simulink library "Valeo_Simulink_Library_EC"  (R2020b)
settings: Solver=ode45  StartTime=0.0  StopTime=10.0  RelTol=1e-3  EnableMultiTasking=on
undefined symbols (not defined in the file): A, B, C, Count_Max, D, InitValue, j, ke, kf, kt, L, Length, MaxIniVal, MaxVal, MinVal, NumBits1, NumBits2, P, p0, Q, R, Simulink_Library, Ts, x0
libraries: $bdroot x9, simulink x4, fixpt_dtprop x4
(part 3 of 4)

== system Valeo_Simulink_Library_EC/Signal_Operations/PosHys ==
  High : Inport
  In : Inport  Port=2
  Low : Inport  Port=3
  DataTypeDuplicate : DataTypeDuplicate  NumInputPorts=3
  Hysteresis : Subsystem  Description=Hysteresis  RTWFileName=sal_math
      settings: RTWSystemCode=Inline  RTWFcnNameOpts=Use subsystem name  RTWFileNameOpts=User specified
  UnitDelay : UnitDelay  SampleTime=-1  HasFrameUpgradeWarning=on
  Out : Outport  VectorParamsAs1DForOutWhenUnconnected=off
  wires:
  Hysteresis/1(Out) -> Out/1, UnitDelay/1
  UnitDelay/1 -> Hysteresis/4(RemainderIN)
  Low/1 -> DataTypeDuplicate/3, Hysteresis/1(Low)
  In/1 -> DataTypeDuplicate/2, Hysteresis/2(In)
  High/1 -> DataTypeDuplicate/1, Hysteresis/3(High)

== system Valeo_Simulink_Library_EC/Signal_Operations/RisingEdge ==
  In : Inport
  LogicalOperator : Logic  Tag=struct('inputs','2','comment',struct('text','','placement',1),'logdata',struct('maxnumvals',inf,'plotchannels',[],'loggingmode',3,'channels',1),'operator','AND','output',struct('variable','','description','','name','$S_$B','address','','class','default','type','Bool','unit',''),'scalingvalid',0,'date',733067.68458487268)  RequirementInfo={} %GIDa_46b4697c_c428_4231_8e35_ed6f95728904  OutDataTypeStr=boolean
  LogicalOperator1 : Logic  Tag=struct('inputs','1','comment',struct('text','','placement',1),'logdata',struct('maxnumvals',inf,'plotchannels',[],'loggingmode',3,'channels',1),'operator','NOT','output',struct('variable','','description','','name','$S_$B','address','','class','default','type','Bool','unit',''),'scalingvalid',0,'date',733067.68458533566)  Operator=NOT  Inputs=1  OutDataTypeStr=boolean
  UnitDelay : UnitDelay  RequirementInfo={} %GIDa_e97586d9_635f_41d8_ab1f_7563d0e0a8e3  InitialCondition=Init  SampleTime=-1  HasFrameUpgradeWarning=on
  Out : Outport  OutDataTypeStr=boolean  VectorParamsAs1DForOutWhenUnconnected=off
  wires:
  UnitDelay/1 -> LogicalOperator/2
  LogicalOperator1/1 -> UnitDelay/1
  LogicalOperator/1 -> Out/1
  In/1 -> LogicalOperator/1, LogicalOperator1/1

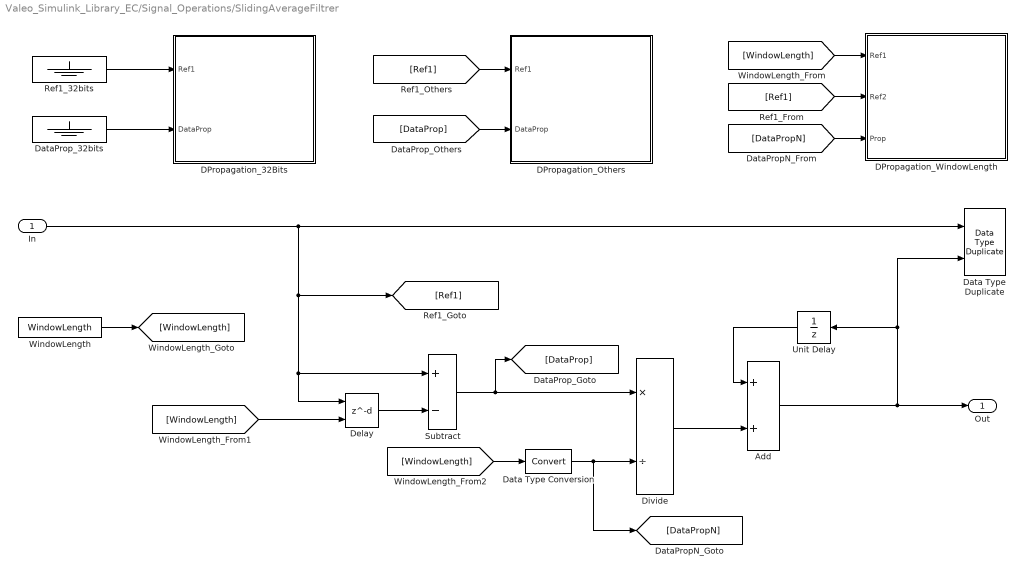
== system Valeo_Simulink_Library_EC/Signal_Operations/SlidingAverageFiltrer ==
  In : Inport
  Add : Sum  OutDataTypeStr=Inherit: Inherit via back propagation  RndMeth=Nearest  SaturateOnIntegerOverflow=on
  DPropagation_32Bits : Subsystem
  DPropagation_Others : Subsystem
  DPropagation_WindowLength : Subsystem
  Data Type Duplicate : DataTypeDuplicate
  Data Type Conversion : DataTypeConversion
  DataProp_32bits : Ground
  Delay : Delay  DelayLengthSource=Input port  DelayLength=Length  DelayLengthUpperLimit=WindowLength  InitialCondition=0
      settings: InputPortMap=u0,p1
  Divide : Product  Inputs=*/  RndMeth=Nearest  OutDataTypeStr=Inherit: Same as first input
  Ref1_32bits : Ground
  Subtract : Sum  Inputs=+-  OutDataTypeStr=Inherit: Inherit via back propagation  RndMeth=Nearest  SaturateOnIntegerOverflow=on
  Unit Delay : UnitDelay  SampleTime=-1  HasFrameUpgradeWarning=on
  WindowLength : Constant  Value=WindowLength  OutDataTypeStr=Inherit: Inherit via back propagation  SampleTime=-1
  Out : Outport  VectorParamsAs1DForOutWhenUnconnected=off
  wires:
  Add/1 -> Out/1, Unit Delay/1, Data Type Duplicate/2
  Delay/1 -> Subtract/2
  Divide/1 -> Add/2
  Unit Delay/1 -> Add/1
  In/1 -> [Ref1], Subtract/1, Delay/1, Data Type Duplicate/1
  Subtract/1 -> [DataProp], Divide/1
  [Ref1] -> DPropagation_Others/1(Ref1)
  [DataProp] -> DPropagation_Others/2(DataProp)
  Ref1_32bits/1 -> DPropagation_32Bits/1(Ref1)
  DataProp_32bits/1 -> DPropagation_32Bits/2(DataProp)
  WindowLength/1 -> [WindowLength]
  [WindowLength] -> Delay/2
  [WindowLength] -> Data Type Conversion/1
  [WindowLength] -> DPropagation_WindowLength/1(Ref1)
  [Ref1] -> DPropagation_WindowLength/2(Ref2)
  Data Type Conversion/1 -> [DataPropN], Divide/2
  [DataPropN] -> DPropagation_WindowLength/3(Prop)

== system Valeo_Simulink_Library_EC/Signal_Operations/TurnOffDelay ==
  In : Inport
  Tdly : Inport  Port=2
  Te : Inport  Port=3
  CheckDly : RelationalOperator  Operator=<  OutDataTypeStr=boolean  RndMeth=Nearest  InputSameDT=on
  Check_Tdly_unsigned : fixpt_dtprop/Data Type Police Unsigned Only
      settings: SourceProductBaseCode=SL
  Check_Te_unsigned : fixpt_dtprop/Data Type Police Unsigned Only
      settings: SourceProductBaseCode=SL
  Divide : Product  Inputs=*/  OutDataTypeStr=uint32  RndMeth=Nearest  SaturateOnIntegerOverflow=on
  Inc : Constant  OutDataTypeStr=Inherit: Inherit via back propagation
  Increment : Sum  InputSameDT=on  OutDataTypeStr=Inherit: Inherit via back propagation  SaturateOnIntegerOverflow=on
  InitialCondition : Subsystem  Description=InitialCondition
  LogicalOperator : Logic  Operator=OR  AllPortsSameDT=off  OutDataTypeStr=boolean
  NewVal : UnitDelay  SampleTime=-1  HasFrameUpgradeWarning=on
  Reset : Constant  Value=0  OutDataTypeStr=Inherit: Inherit via back propagation
  ResetSwitch : Switch  Criteria=u2 ~= 0  InputSameDT=on
  StartDelay : UnitDelay  SampleTime=-1  HasFrameUpgradeWarning=on
  Out : Outport  VectorParamsAs1DForOutWhenUnconnected=off
  wires:
  LogicalOperator/1 -> Out/1
  Reset/1 -> ResetSwitch/1
  ResetSwitch/1 -> Increment/1, CheckDly/1
  Increment/1 -> NewVal/1
  CheckDly/1 -> LogicalOperator/1
  In/1 -> LogicalOperator/2, InitialCondition/1(CheckDir), StartDelay/1
  NewVal/1 -> InitialCondition/3(NewVal)
  InitialCondition/1(CalcVal) -> ResetSwitch/3
  StartDelay/1 -> ResetSwitch/2
  Divide/1 -> CheckDly/2, InitialCondition/2(Tdly)
  Te/1 -> Check_Te_unsigned/1, Divide/2
  Tdly/1 -> Check_Tdly_unsigned/1, Divide/1
  Inc/1 -> Increment/2

== system Valeo_Simulink_Library_EC/Signal_Operations/TurnOnDelay ==
  In : Inport
  Tdly : Inport  Port=2
  Te : Inport  Port=3
  CheckDly : RelationalOperator  OutDataTypeStr=boolean  RndMeth=Nearest  InputSameDT=on
  Check_Tdly_unsigned : fixpt_dtprop/Data Type Police Unsigned Only
      settings: SourceProductBaseCode=SL
  Check_Te_unsigned : fixpt_dtprop/Data Type Police Unsigned Only
      settings: SourceProductBaseCode=SL
  Divide : Product  Inputs=*/  OutDataTypeStr=uint32  SaturateOnIntegerOverflow=on
  Inc : Constant  OutDataTypeStr=Inherit: Inherit via back propagation
  Increment : Sum  InputSameDT=on  OutDataTypeStr=Inherit: Inherit via back propagation  RndMeth=Simplest  SaturateOnIntegerOverflow=on
  InitialCondition : Subsystem  Description=InitialCondition
  InitialDelayl : UnitDelay  InitialCondition=1  SampleTime=-1  HasFrameUpgradeWarning=on
  LogicalOperator : Logic  AllPortsSameDT=off  OutDataTypeStr=boolean
  NewVal : UnitDelay  SampleTime=-1  HasFrameUpgradeWarning=on
  Reset : Constant  Value=0  OutDataTypeStr=Inherit: Inherit via back propagation
  ResetSwitch : Switch  Criteria=u2 ~= 0  InputSameDT=on
  Out : Outport  VectorParamsAs1DForOutWhenUnconnected=off
  wires:
  InitialDelayl/1 -> ResetSwitch/2
  LogicalOperator/1 -> Out/1
  ResetSwitch/1 -> Increment/1, CheckDly/1
  Increment/1 -> NewVal/1
  CheckDly/1 -> LogicalOperator/1
  NewVal/1 -> InitialCondition/1(NewVal)
  In/1 -> LogicalOperator/2, InitialCondition/3(CheckDir), InitialDelayl/1
  InitialCondition/1(CalcVal) -> ResetSwitch/1
  Reset/1 -> ResetSwitch/3
  Tdly/1 -> Divide/1, Check_Tdly_unsigned/1
  Te/1 -> Divide/2, Check_Te_unsigned/1
  Divide/1 -> InitialCondition/2(Tdly), CheckDly/2
  Inc/1 -> Increment/2

== system Valeo_Simulink_Library_EC/Signal_Operations/VSL_ClarkTransformation_EC_Blk ==
  A : Inport  PortDimensions=1
  B : Inport  Port=2  PortDimensions=1
  C : Inport  Port=3  PortDimensions=1
  Calculation : Subsystem  Description=Calculations for clarke transfromation  RequirementInfo={} %GIDa_91c9902b_4297_47d8_bcc7_839692c95106
  datatype_protection : Subsystem  Description=forcing input and output to have the same data type  RequirementInfo={} %GIDa_ba0677aa_132e_4dc0_8af7_6cee4e109de7
  Alpha : Outport  RequirementInfo={} %GIDa_2f11082c_73d3_4ed4_8929_d03a8ab0ed51  PortDimensions=1  VectorParamsAs1DForOutWhenUnconnected=off
  Beta : Outport  RequirementInfo={} %GIDa_b2cc2919_a1d0_479c_944a_1162b348937b  Port=2  PortDimensions=1  VectorParamsAs1DForOutWhenUnconnected=off
  wires:
  B/1 -> [B]  "B"
  A/1 -> [A]  "A"
  C/1 -> [C]  "C"
  [A] -> Calculation/1(A)
  [B] -> Calculation/2(B)
  [C] -> Calculation/3(C)
  datatype_protection/1(Alpha) -> Alpha/1
  datatype_protection/2(Beta) -> Beta/1
  Calculation/1(Alpha) -> datatype_protection/1(Alpha_temp)
  Calculation/2(Beta) -> datatype_protection/2(Beta_temp)
  [A] -> datatype_protection/3(A)
  [B] -> datatype_protection/4(B)
  [C] -> datatype_protection/5(C)

== system Valeo_Simulink_Library_EC/Signal_Operations/VSL_InverseClarkTransformation_EC_Blk ==
  Alpha : Inport
  Beta : Inport  Port=2
  Calculations : Subsystem  Description=claclulations of Inverse clarke transform
  "DataTypeProtection " : Subsystem  Description=make sure all inputs and outputs have the same datatype
  A : Outport  VectorParamsAs1DForOutWhenUnconnected=off
  B : Outport  Port=2  VectorParamsAs1DForOutWhenUnconnected=off
  C : Outport  Port=3  VectorParamsAs1DForOutWhenUnconnected=off
  wires:
  Calculations/1(A) -> "DataTypeProtection "/1(A_t)
  Calculations/2(B) -> "DataTypeProtection "/2(B_t)
  Calculations/3(C) -> "DataTypeProtection "/3(C_t)
  "DataTypeProtection "/1(A) -> A/1
  "DataTypeProtection "/2(B) -> B/1
  "DataTypeProtection "/3(C) -> C/1
  [Alpha] -> Calculations/1(Alpha)
  [Beta] -> Calculations/2(Beta)
  [Alpha] -> "DataTypeProtection "/4(Alpha)
  [Beta] -> "DataTypeProtection "/5(Beta)
  Alpha/1 -> [Alpha]
  Beta/1 -> [Beta]

== system Valeo_Simulink_Library_EC/Signal_Operations/VSL_InverseParkTransformation_EC_Blk ==
  D : Inport
  Q : Inport  Port=2
  Sin : Inport  Port=3
  Cos : Inport  Port=4
  Calculation : Subsystem  Description=This Block is transforming dq axies with d axis aligned with Phase A into alpha-beta axises
      settings: RTWFcnNameOpts=Use subsystem name
  dataTypeProtection : Subsystem  Description=make sure inputs and outputs have the same data type
  Alpha : Outport  VectorParamsAs1DForOutWhenUnconnected=off
  Beta : Outport  Port=2  VectorParamsAs1DForOutWhenUnconnected=off
  wires:
  [Cos] -> dataTypeProtection/6(Cos)
  [Sin] -> dataTypeProtection/5(Sin)
  [Q] -> dataTypeProtection/4(Q)
  [D] -> dataTypeProtection/3(D)
  dataTypeProtection/1(Alpha) -> Alpha/1  "Alpha"
  dataTypeProtection/2(Beta) -> Beta/1  "Beta"
  [Cos] -> Calculation/3(cos)
  [Sin] -> Calculation/2(sin)
  Cos/1 -> [Cos]
  Sin/1 -> [Sin]
  [Q] -> Calculation/4(Q)
  [D] -> Calculation/1(D)
  D/1 -> [D]
  Q/1 -> [Q]
  Calculation/2(Beta) -> dataTypeProtection/2(beta_t)
  Calculation/1(Alpha) -> dataTypeProtection/1(alpha_t)

== system Valeo_Simulink_Library_EC/Signal_Operations/VSL_ParkTransformation_Blk ==
  Alpha : Inport
  Beta : Inport  Port=2
  Sin : Inport  Port=3
  Cos : Inport  Port=4
  Calculation : Subsystem  Description=This Block is transforming alpha-beta axises into dq axies with d axie aligned with Phase A
      settings: RTWSystemCode=Nonreusable function  RTWFcnNameOpts=Use subsystem name
  DataTypeProtection : Subsystem  Description=make sure all inputs and outputs have the sane data type
  D : Outport  VectorParamsAs1DForOutWhenUnconnected=off
  Q : Outport  Port=2  VectorParamsAs1DForOutWhenUnconnected=off
  wires:
  Beta/1 -> [beta]
  Alpha/1 -> [alpha]
  [alpha] -> Calculation/1(alpha)
  [beta] -> Calculation/4(beta)
  Calculation/1(d) -> DataTypeProtection/1(d_t)  "D"
  Calculation/2(q) -> DataTypeProtection/2(q_t)  "Q"
  Sin/1 -> [sin]
  Cos/1 -> [cos]
  [sin] -> Calculation/2(sin)
  [cos] -> Calculation/3(cos)
  DataTypeProtection/1(D) -> D/1
  DataTypeProtection/2(Q) -> Q/1
  [alpha] -> DataTypeProtection/3(Alpha)
  [beta] -> DataTypeProtection/4(Beta)
  [sin] -> DataTypeProtection/5(Sin)
  [cos] -> DataTypeProtection/6(Cos)

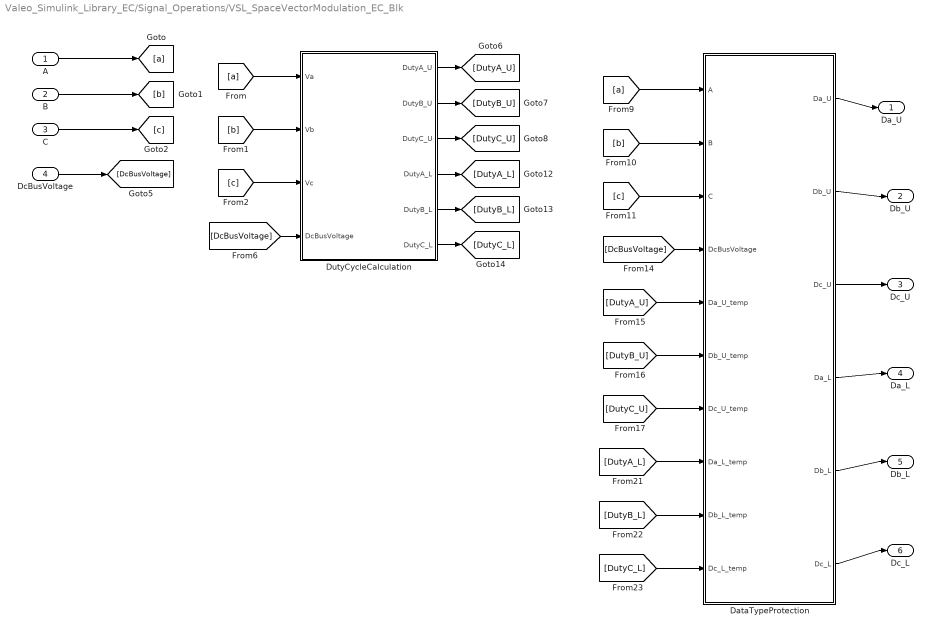
== system Valeo_Simulink_Library_EC/Signal_Operations/VSL_SpaceVectorModulation_EC_Blk ==
  A : Inport
  B : Inport  Port=2
  C : Inport  Port=3
  DcBusVoltage : Inport  Port=4
  DataTypeProtection : Subsystem  Description=applying the data type protection
  DutyCycleCalculation : Subsystem  Description=Calculate the duty cycle for every phase
  Da_U : Outport  VectorParamsAs1DForOutWhenUnconnected=off
  Db_U : Outport  Port=2  VectorParamsAs1DForOutWhenUnconnected=off
  Dc_U : Outport  Port=3  VectorParamsAs1DForOutWhenUnconnected=off
  Da_L : Outport  Port=4  VectorParamsAs1DForOutWhenUnconnected=off
  Db_L : Outport  Port=5  VectorParamsAs1DForOutWhenUnconnected=off
  Dc_L : Outport  Port=6  VectorParamsAs1DForOutWhenUnconnected=off
  wires:
  DataTypeProtection/6(Dc_L) -> Dc_L/1
  DataTypeProtection/5(Db_L) -> Db_L/1
  DataTypeProtection/4(Da_L) -> Da_L/1
  DataTypeProtection/3(Dc_U) -> Dc_U/1
  DataTypeProtection/2(Db_U) -> Db_U/1
  DataTypeProtection/1(Da_U) -> Da_U/1
  [DutyC_L] -> DataTypeProtection/10(Dc_L_temp)
  [DutyA_L] -> DataTypeProtection/8(Da_L_temp)
  [DutyB_L] -> DataTypeProtection/9(Db_L_temp)
  [DutyC_U] -> DataTypeProtection/7(Dc_U_temp)
  [DutyB_U] -> DataTypeProtection/6(Db_U_temp)
  DutyCycleCalculation/4(DutyA_L) -> [DutyA_L]
  DutyCycleCalculation/5(DutyB_L) -> [DutyB_L]
  DutyCycleCalculation/6(DutyC_L) -> [DutyC_L]
  [c] -> DutyCycleCalculation/3(Vc)
  [b] -> DutyCycleCalculation/2(Vb)
  [a] -> DutyCycleCalculation/1(Va)
  B/1 -> [b]
  C/1 -> [c]
  A/1 -> [a]
  DcBusVoltage/1 -> [DcBusVoltage]
  [DcBusVoltage] -> DutyCycleCalculation/4(DcBusVoltage)
  [a] -> DataTypeProtection/1(A)
  [b] -> DataTypeProtection/2(B)
  [c] -> DataTypeProtection/3(C)
  [DcBusVoltage] -> DataTypeProtection/4(DcBusVoltage)
  DutyCycleCalculation/1(DutyA_U) -> [DutyA_U]
  DutyCycleCalculation/2(DutyB_U) -> [DutyB_U]
  DutyCycleCalculation/3(DutyC_U) -> [DutyC_U]
  [DutyA_U] -> DataTypeProtection/5(Da_U_temp)

== system Valeo_Simulink_Library_EC/Utilities/EventToVar ==
  Evt : Inport
  Constant1 : Constant  Value=0  OutDataTypeStr=boolean  SampleTime=-1
  Constant2 : Constant  OutDataTypeStr=boolean  SampleTime=-1
  Function-Call Subsystem : Subsystem  Description=|  TreatAsAtomicUnit=on
      | Function-Call
      | Subsystem
  Logical Operator1 : Logic  Tag=AM,Std,Inputs,1;CMP,Operator,Inputs;  Operator=NOT  Inputs=1  AllPortsSameDT=off  OutDataTypeStr=boolean
  Relational Operator : RelationalOperator  Operator=~=  OutDataTypeStr=boolean  RndMeth=Nearest
  Switch : Switch  Criteria=u2 ~= 0
  Unit Delay1 : UnitDelay  SampleTime=-1  HasFrameUpgradeWarning=on
  Unit Delay2 : UnitDelay  SampleTime=-1  HasFrameUpgradeWarning=on
  Var : Outport  VectorParamsAs1DForOutWhenUnconnected=off
  wires:
  Logical Operator1/1 -> Relational Operator/1, Unit Delay1/1
  Switch/1 -> Var/1
  Relational Operator/1 -> Switch/2
  Constant1/1 -> Switch/3
  Constant2/1 -> Switch/1
  Unit Delay1/1 -> Relational Operator/2
  Function-Call Subsystem/1(out) -> Logical Operator1/1, Unit Delay2/1
  Unit Delay2/1 -> Function-Call Subsystem/1(in)
  Evt/1 -> Function-Call Subsystem/Trigger

== system Valeo_Simulink_Library_EC/Utilities/ScribeInfo ==

== system Valeo_Simulink_Library_EC/Math_Operations/VSL_DynamicSecureDivision_EC_Blk/Calculation ==
  Num : Inport  PortDimensions=1
  Den : Inport  Port=2  PortDimensions=1
  Positive_Inf : Inport  Port=3  PortDimensions=1
  Negative_Inf : Inport  Port=4  PortDimensions=1
  Nan : Inport  Port=5  PortDimensions=1
  ZeroBand_Den : Inport  Port=6  PortDimensions=1
  ZeroBand_Num : Inport  Port=7  PortDimensions=1
  DecisionLogic : Subsystem  Description=Decision logic for dynamic secure division. this block is performing secure division with Positive_inf, Negative_inf, Nan is dynamic in run time
  Divide : Subsystem  TreatAsAtomicUnit=on
  Merge : Merge  InitialOutput=0
  Output : Outport  VectorParamsAs1DForOutWhenUnconnected=off
  wires:
  ZeroBand_Num/1 -> DecisionLogic/7(ZeroBand_Num)
  ZeroBand_Den/1 -> DecisionLogic/6(ZeroBand_Den)
  Positive_Inf/1 -> DecisionLogic/3(Positive_Inf)
  Negative_Inf/1 -> DecisionLogic/4(Negative_Inf)
  Nan/1 -> DecisionLogic/5(Nan)
  DecisionLogic/1(Out) -> Merge/1
  DecisionLogic/2(Divide) -> Divide/Trigger
  Merge/1 -> Output/1
  Divide/1(output) -> Merge/2
  Den/1 -> DecisionLogic/2(Den), Divide/2(Den)
  Num/1 -> DecisionLogic/1(Num), Divide/1(Num)

== system Valeo_Simulink_Library_EC/Math_Operations/VSL_DynamicSecureDivision_EC_Blk/datatype_protection ==
  Output_Temp : Inport  PortDimensions=1
  P_inf : Inport  Port=2  PortDimensions=1
  N_inf : Inport  Port=3  PortDimensions=1
  Nan : Inport  Port=4  PortDimensions=1
  Den : Inport  Port=5  PortDimensions=1
  ZeroBand_Den : Inport  Port=6  PortDimensions=1
  Num : Inport  Port=7  PortDimensions=1
  ZeroBand_num : Inport  Port=8  PortDimensions=1
  Data Type Duplicate : DataTypeDuplicate  RequirementInfo={} %GIDa_59c1057f_2c2c_4435_a6e2_f9e4eb9c7f02  NumInputPorts=4
  Data Type Duplicate1 : DataTypeDuplicate  RequirementInfo={} %GIDa_59c1057f_2c2c_4435_a6e2_f9e4eb9c7f02
  Data Type Duplicate2 : DataTypeDuplicate  RequirementInfo={} %GIDa_59c1057f_2c2c_4435_a6e2_f9e4eb9c7f02
  Output : Outport  VectorParamsAs1DForOutWhenUnconnected=off
  wires:
  Num/1 -> Data Type Duplicate2/1
  ZeroBand_num/1 -> Data Type Duplicate2/2
  Den/1 -> Data Type Duplicate1/1
  ZeroBand_Den/1 -> Data Type Duplicate1/2
  Nan/1 -> Data Type Duplicate/4
  N_inf/1 -> Data Type Duplicate/3
  P_inf/1 -> Data Type Duplicate/2
  Output_Temp/1 -> Data Type Duplicate/1, Output/1

== system Valeo_Simulink_Library_EC/Plant Models/Actuators/BLDC ==
  Vs : Inport
  TL : Inport  Port=2
  BLDC motor Block : Subsystem
  inverter : Subsystem
  Te : Outport  VectorParamsAs1DForOutWhenUnconnected=off
  omega(rad/sec) : Outport  Port=2  VectorParamsAs1DForOutWhenUnconnected=off
  Position : Outport  Port=3  VectorParamsAs1DForOutWhenUnconnected=off
  i_abc : Outport  Port=4  VectorParamsAs1DForOutWhenUnconnected=off
  wires:
  BLDC motor Block/4(B_EMF) -> inverter/3(B_EMF)
  BLDC motor Block/1(Te) -> Te/1
  BLDC motor Block/3(Position) -> Position/1, inverter/1(POS)
  inverter/1("Uab, Ubc") -> BLDC motor Block/1(" Uab,Ubc")
  TL/1 -> BLDC motor Block/2(Tl)
  BLDC motor Block/5(i_abc) -> inverter/4(i_abc), i_abc/1
  Vs/1 -> inverter/2(Vs)
  BLDC motor Block/2(Omega) -> omega(rad/sec)/1  "omega(rad/sec)"

== system Valeo_Simulink_Library_EC/Signal_Operations/Debouncing_Blk/Else ==
  In : Inport
  Action Port : ActionPort
  Signal Conversion : SignalConversion  OverrideOpt=off
  Out : Outport  VectorParamsAs1DForOutWhenUnconnected=off
  wires:
  In/1 -> Signal Conversion/1
  Signal Conversion/1 -> Out/1

== system Valeo_Simulink_Library_EC/Signal_Operations/Debouncing_Blk/Turn_OFF ==
  Action Port : ActionPort
  Constant1 : Constant  Value=0  OutDataTypeStr=uint8  SampleTime=-1
  Constant3 : Constant  Value=0  OutDataTypeStr=boolean  SampleTime=-1
  Counter : Outport  VectorParamsAs1DForOutWhenUnconnected=off
  Out : Outport  Port=2  VectorParamsAs1DForOutWhenUnconnected=off
  wires:
  Constant3/1 -> Out/1
  Constant1/1 -> Counter/1

== system Valeo_Simulink_Library_EC/Signal_Operations/Debouncing_Blk/Turn_ON ==
  Action Port : ActionPort
  Constant3 : Constant  Value=0  OutDataTypeStr=uint8  SampleTime=-1
  Constant4 : Constant  OutDataTypeStr=boolean  SampleTime=-1
  Out : Outport  VectorParamsAs1DForOutWhenUnconnected=off
  Counter : Outport  Port=2  VectorParamsAs1DForOutWhenUnconnected=off
  wires:
  Constant4/1 -> Out/1
  Constant3/1 -> Counter/1

== system Valeo_Simulink_Library_EC/Signal_Operations/KalmanFilter_single/Correct ==
  u : Inport
  Yk : Inport  Port=2
  Pk_priori : Inport  Port=3
  Xk_priori : Inport  Port=4
  Constant1 : Constant  Value=C  VectorParams1D=off  OutDataTypeStr=single
  Constant3 : Constant  Value=R  VectorParams1D=off  OutDataTypeStr=single
  K_opt : Subsystem
  P_k : Subsystem
  X_k : Subsystem
  Pk : Outport  OutDataTypeStr=single  InitialOutput=0  VectorParamsAs1DForOutWhenUnconnected=off
  Xk : Outport  Port=2  OutDataTypeStr=single  InitialOutput=3  VectorParamsAs1DForOutWhenUnconnected=off
  wires:
  Pk_priori/1 -> P_k/1(Pk_priori), K_opt/1(Pk_priori)
  Constant3/1 -> [R]
  Yk/1 -> X_k/2(Yk)
  Xk_priori/1 -> X_k/3(Xk_priori)
  u/1 -> X_k/4(u)
  X_k/1(Xk) -> Xk/1
  Constant1/1 -> [C]
  [C] -> X_k/5(C)
  K_opt/1(K_optimal) -> X_k/1(K_optimal), P_k/2(In2)
  P_k/1(Pk) -> Pk/1
  [R] -> P_k/3(R)
  [C] -> P_k/4(C)
  [R] -> K_opt/2(R)
  [C] -> K_opt/3(C)

== system Valeo_Simulink_Library_EC/Signal_Operations/KalmanFilter_single/Predict ==
  u : Inport
  Pk-1 : Inport  Port=2
  Xk-1 : Inport  Port=3
  Add : Sum
  Add1 : Sum
  Constant : Constant  Value=A  VectorParams1D=off  OutDataTypeStr=single
  Constant1 : Constant  Value=Q  VectorParams1D=off  OutDataTypeStr=single
  Constant2 : Constant  Value=B  VectorParams1D=off  OutDataTypeStr=single
  Math Function : Math  Operator=transpose  SignedPower=on  SaturateOnIntegerOverflow=on
  Product : Product  Inputs=3  Multiplication=Matrix(*)
  Product1 : Product  Inputs=**  Multiplication=Matrix(*)  RndMeth=Zero
  Product2 : Product  Inputs=**  Multiplication=Matrix(*)  RndMeth=Zero
  Pk_priori : Outport  OutDataTypeStr=single  VectorParamsAs1DForOutWhenUnconnected=off
  Xk_priori : Outport  Port=2  OutDataTypeStr=single  VectorParamsAs1DForOutWhenUnconnected=off
  wires:
  Constant2/1 -> Product2/1
  Math Function/1 -> Product/3
  Constant/1 -> Product/1, Product1/1, Math Function/1
  Product/1 -> Add1/2
  Pk-1/1 -> Product/2
  Product1/1 -> Add/1
  Xk-1/1 -> Product1/2
  u/1 -> Product2/2
  Product2/1 -> Add/2
  Add1/1 -> Pk_priori/1
  Constant1/1 -> Add1/1
  Add/1 -> Xk_priori/1

== system Valeo_Simulink_Library_EC/Signal_Operations/NegHys/Hysteresis ==
  Low : Inport
  In : Inport  Port=2
  High : Inport  Port=3
  RemainderIN : Inport  Port=4
  Constant : Constant  Value=0  OutDataTypeStr=boolean
  Constant1 : Constant  OutDataTypeStr=boolean
  RelationalOperator3 : RelationalOperator  OutDataTypeStr=boolean  RndMeth=Nearest  InputSameDT=on
  RelationalOperator4 : RelationalOperator  OutDataTypeStr=boolean  RndMeth=Nearest  InputSameDT=on
  Switch : Switch  Criteria=u2 ~= 0  OutDataTypeStr=Inherit: Inherit via back propagation  InputSameDT=on
  Switch1 : Switch  Criteria=u2 ~= 0  OutDataTypeStr=Inherit: Inherit via back propagation  InputSameDT=on
  Out : Outport  VectorParamsAs1DForOutWhenUnconnected=off
  wires:
  RemainderIN/1 -> Switch1/3
  Switch/1 -> Out/1
  Switch1/1 -> Switch/3
  RelationalOperator4/1 -> Switch1/2
  Constant/1 -> Switch1/1
  RelationalOperator3/1 -> Switch/2
  Constant1/1 -> Switch/1
  Low/1 -> RelationalOperator3/1
  High/1 -> RelationalOperator4/2
  In/1 -> RelationalOperator4/1, RelationalOperator3/2

== system Valeo_Simulink_Library_EC/Signal_Operations/PosHys/Hysteresis ==
  Low : Inport
  In : Inport  Port=2
  High : Inport  Port=3
  RemainderIN : Inport  Port=4
  Constant : Constant  OutDataTypeStr=boolean
  Constant1 : Constant  Value=0  OutDataTypeStr=boolean
  RelationalOperator3 : RelationalOperator  OutDataTypeStr=boolean  RndMeth=Nearest  InputSameDT=on
  RelationalOperator4 : RelationalOperator  OutDataTypeStr=boolean  RndMeth=Nearest  InputSameDT=on
  Switch : Switch  Criteria=u2 ~= 0  OutDataTypeStr=Inherit: Inherit via back propagation  InputSameDT=on
  Switch1 : Switch  Criteria=u2 ~= 0  OutDataTypeStr=Inherit: Inherit via back propagation  InputSameDT=on
  Out : Outport  VectorParamsAs1DForOutWhenUnconnected=off
  wires:
  In/1 -> RelationalOperator3/2, RelationalOperator4/1
  High/1 -> RelationalOperator4/2
  Low/1 -> RelationalOperator3/1
  Constant1/1 -> Switch/1
  RelationalOperator3/1 -> Switch/2
  Constant/1 -> Switch1/1
  RelationalOperator4/1 -> Switch1/2
  Switch1/1 -> Switch/3
  Switch/1 -> Out/1
  RemainderIN/1 -> Switch1/3

== system Valeo_Simulink_Library_EC/Signal_Operations/SlidingAverageFiltrer/DPropagation_32Bits ==
  Ref1 : Inport
  DataProp : Inport  Port=2
  Data Type Propagation : simulink/Signal Attributes/Data Type Propagation  PropDataType=fixdt(1, 16)  IfRefDouble=double  IfRefSingle=single  IsSigned=TRUE  NumBitsBase=NumBits1  NumBitsMult=1  NumBitsAdd=0  NumBitsAllowFinal=8:32  PropScaling=2^-10  ValuesUsedBestPrec=[5 -7]  SlopeBase=Slope1  SlopeMult=1  SlopeAdd=0  BiasBase=Bias1  BiasMult=1  BiasAdd=0
      settings: SourceProductBaseCode=SL
  wires:
  Ref1/1 -> Data Type Propagation/2, Data Type Propagation/1
  DataProp/1 -> Data Type Propagation/3

== system Valeo_Simulink_Library_EC/Signal_Operations/SlidingAverageFiltrer/DPropagation_Others ==
  Ref1 : Inport
  DataProp : Inport  Port=2
  Data Type Propagation : simulink/Signal Attributes/Data Type Propagation  PropDataType=fixdt(1, 16)  IfRefDouble=double  IfRefSingle=single  IsSigned=TRUE  NumBitsBase=NumBits1+NumBits2  NumBitsMult=1  NumBitsAdd=0  NumBitsAllowFinal=8:32  PropScaling=2^-10  ValuesUsedBestPrec=[5 -7]  SlopeBase=Slope1  SlopeMult=1  SlopeAdd=0  BiasBase=Bias1  BiasMult=1  BiasAdd=0
      settings: SourceProductBaseCode=SL
  wires:
  DataProp/1 -> Data Type Propagation/3
  Ref1/1 -> Data Type Propagation/2, Data Type Propagation/1

== system Valeo_Simulink_Library_EC/Signal_Operations/SlidingAverageFiltrer/DPropagation_WindowLength ==
  Ref1 : Inport
  Ref2 : Inport  Port=2
  Prop : Inport  Port=3
  Data Type Propagation : simulink/Signal Attributes/Data Type Propagation  PropDataType=fixdt(1, 16)  IfRefDouble=double  IfRefSingle=single  IsSigned=FALSE  NumBitsBase=NumBits1  NumBitsMult=1  NumBitsAdd=0  NumBitsAllowFinal=8:32  PropScaling=2^-10  ValuesUsedBestPrec=[5 -7]  SlopeBase=Slope1  SlopeMult=1  SlopeAdd=0  BiasBase=Bias1  BiasMult=1  BiasAdd=0
      settings: SourceProductBaseCode=SL
  wires:
  Ref1/1 -> Data Type Propagation/1
  Ref2/1 -> Data Type Propagation/2
  Prop/1 -> Data Type Propagation/3

== system Valeo_Simulink_Library_EC/Signal_Operations/TurnOffDelay/InitialCondition ==
  CheckDir : Inport
  Tdly : Inport  Port=2
  NewVal : Inport  Port=3
  LogicalOperator1 : Logic  Operator=OR  AllPortsSameDT=off  OutDataTypeStr=boolean
  NewVal1 : UnitDelay  InitialCondition=1  SampleTime=-1  HasFrameUpgradeWarning=on
  Reset : Constant  Value=0  OutDataTypeStr=boolean
  Switch : Switch  Criteria=u2 ~= 0  InputSameDT=on
  CalcVal : Outport  VectorParamsAs1DForOutWhenUnconnected=off
  wires:
  NewVal/1 -> Switch/3
  Tdly/1 -> Switch/1
  NewVal1/1 -> LogicalOperator1/2
  Reset/1 -> NewVal1/1
  LogicalOperator1/1 -> Switch/2
  CheckDir/1 -> LogicalOperator1/1
  Switch/1 -> CalcVal/1

== system Valeo_Simulink_Library_EC/Signal_Operations/TurnOnDelay/InitialCondition ==
  NewVal : Inport
  Tdly : Inport  Port=2
  CheckDir : Inport  Port=3
  LogicalOperator : Logic  Operator=NOT  AllPortsSameDT=off  OutDataTypeStr=boolean
  LogicalOperator1 : Logic  Operator=OR  AllPortsSameDT=off  OutDataTypeStr=boolean
  NewVal1 : UnitDelay  SampleTime=-1  HasFrameUpgradeWarning=on
  Reset : Constant  OutDataTypeStr=boolean
  Switch : Switch  Criteria=u2 ~= 0  InputSameDT=on
  CalcVal : Outport  VectorParamsAs1DForOutWhenUnconnected=off
  wires:
  NewVal/1 -> Switch/1
  NewVal1/1 -> LogicalOperator1/2
  Reset/1 -> NewVal1/1
  LogicalOperator1/1 -> Switch/2
  Switch/1 -> CalcVal/1
  Tdly/1 -> Switch/3
  CheckDir/1 -> LogicalOperator/1
  LogicalOperator/1 -> LogicalOperator1/1

== system Valeo_Simulink_Library_EC/Signal_Operations/VSL_ClarkTransformation_EC_Blk/Calculation ==
  A : Inport
  B : Inport  Port=2
  C : Inport  Port=3
  Add : Sum  RequirementInfo={} %GIDa_afe2c577_734f_4faf_b375_0ef20aeeab01  Inputs=+++  OutDataTypeStr=Inherit: Inherit via back propagation  RndMeth=Simplest
  Add1 : Sum  RequirementInfo={} %GIDa_b8b12de4_a1c3_404a_a9d1_be098477dac5  OutDataTypeStr=Inherit: Inherit via back propagation  RndMeth=Simplest
  Const_2Over3 : Gain  Description=gain of 0.666 as 0.666  RequirementInfo={} %GIDa_120f91ab_5e07_4588_9a66_f8fa17d7ebbb  Gain=0.6667  OutDataTypeStr=Inherit: Inherit via back propagation  RndMeth=Simplest  ParamDataTypeStr=Inherit: Same as input
  Const_Neg1Over3 : Gain  Description=gain of -.333 as -.333  RequirementInfo={} %GIDa_cbff4a56_eba5_4d1b_82e9_2b912c46c30a  Gain=-.3333  OutDataTypeStr=Inherit: Inherit via back propagation  RndMeth=Simplest  ParamDataTypeStr=Inherit: Same as input
  Const_Neg1Over3_2 : Gain  Description=gain of -.333 as -.333  RequirementInfo={} %GIDa_82831831_6244_46f4_8700_983a6e4d662e  Gain=-.3333  OutDataTypeStr=Inherit: Inherit via back propagation  RndMeth=Simplest  ParamDataTypeStr=Inherit: Same as input
  Const_NegSqrt3Over3 : Gain  Description=gain of -.577 as -sqrt(3)/3  RequirementInfo={} %GIDa_a4218fb9_5262_4d86_8cc2_5cb31cf1db53  Gain=-.5773  OutDataTypeStr=Inherit: Inherit via back propagation  RndMeth=Simplest  ParamDataTypeStr=Inherit: Same as input
  Const_Sqrt3Over2 : Gain  Description=gain of .577 as sqrt(3)/3  RequirementInfo={} %GIDa_f78375a3_f7cc_4d79_b4c2_30115ac82f8c  Gain=.5773  OutDataTypeStr=Inherit: Inherit via back propagation  RndMeth=Simplest  ParamDataTypeStr=Inherit: Same as input
  Alpha : Outport  VectorParamsAs1DForOutWhenUnconnected=off
  Beta : Outport  Port=2  VectorParamsAs1DForOutWhenUnconnected=off
  wires:
  Const_NegSqrt3Over3/1 -> Add1/2
  Const_2Over3/1 -> Add/2
  Const_Neg1Over3/1 -> Add/1
  B/1 -> Const_Sqrt3Over2/1, Const_Neg1Over3/1
  Const_Neg1Over3_2/1 -> Add/3
  Add/1 -> Alpha/1  "Alpha"
  A/1 -> Const_2Over3/1
  C/1 -> Const_Neg1Over3_2/1, Const_NegSqrt3Over3/1
  Add1/1 -> Beta/1  "Beta"
  Const_Sqrt3Over2/1 -> Add1/1

== system Valeo_Simulink_Library_EC/Signal_Operations/VSL_ClarkTransformation_EC_Blk/datatype_protection ==
  Alpha_temp : Inport  PortDimensions=1
  Beta_temp : Inport  Port=2  PortDimensions=1
  A : Inport  Port=3  PortDimensions=1
  B : Inport  Port=4  PortDimensions=1
  C : Inport  Port=5  PortDimensions=1
  Data Type Duplicate : DataTypeDuplicate  RequirementInfo={} %GIDa_59c1057f_2c2c_4435_a6e2_f9e4eb9c7f02  NumInputPorts=5
  Alpha : Outport  VectorParamsAs1DForOutWhenUnconnected=off
  Beta : Outport  Port=2  VectorParamsAs1DForOutWhenUnconnected=off
  wires:
  A/1 -> Data Type Duplicate/2
  B/1 -> Data Type Duplicate/3
  C/1 -> Data Type Duplicate/4
  Beta_temp/1 -> Beta/1, Data Type Duplicate/5
  Alpha_temp/1 -> Alpha/1, Data Type Duplicate/1

== system Valeo_Simulink_Library_EC/Signal_Operations/VSL_InverseClarkTransformation_EC_Blk/Calculations ==
  Alpha : Inport
  Beta : Inport  Port=2
  Add1 : Sum  OutDataTypeStr=Inherit: Inherit via back propagation  RndMeth=Simplest
  Add2 : Sum  OutDataTypeStr=Inherit: Inherit via back propagation  RndMeth=Simplest
  Const_1Over2 : Gain  Description=-1/2  Gain=-0.5  OutDataTypeStr=Inherit: Inherit via back propagation  RndMeth=Simplest  ParamDataTypeStr=Inherit: Same as input
      settings: AttributesFormatString=%<ShowName>
  Const_NegSqrt3Over2 : Gain  Description=-Sqrt(3)/3  Gain=-0.8660  OutDataTypeStr=Inherit: Inherit via back propagation  RndMeth=Simplest  ParamDataTypeStr=Inherit: Same as input
      settings: AttributesFormatString=%<ShowName>
  Const_Sqrt3Over2 : Gain  Description=Sqrt(3)/3  Gain=0.8660  OutDataTypeStr=Inherit: Inherit via back propagation  RndMeth=Simplest  ParamDataTypeStr=Inherit: Same as input
      settings: AttributesFormatString=%<ShowName>
  Signal Conversion : SignalConversion  OverrideOpt=off
  A : Outport  VectorParamsAs1DForOutWhenUnconnected=off
  B : Outport  Port=2  VectorParamsAs1DForOutWhenUnconnected=off
  C : Outport  Port=3  VectorParamsAs1DForOutWhenUnconnected=off
  wires:
  Const_NegSqrt3Over2/1 -> Add2/1
  Add2/1 -> C/1  "C"
  Signal Conversion/1 -> A/1  "A"
  Const_Sqrt3Over2/1 -> Add1/1
  Const_1Over2/1 -> Add1/2, Add2/2
  Add1/1 -> B/1  "B"
  Beta/1 -> Const_Sqrt3Over2/1, Const_NegSqrt3Over2/1
  Alpha/1 -> Signal Conversion/1, Const_1Over2/1

== system Valeo_Simulink_Library_EC/Signal_Operations/VSL_InverseClarkTransformation_EC_Blk/DataTypeProtection  ==
  A_t : Inport
  B_t : Inport  Port=2
  C_t : Inport  Port=3
  Alpha : Inport  Port=4
  Beta : Inport  Port=5
  Data Type Duplicate : DataTypeDuplicate  NumInputPorts=5
  A : Outport  VectorParamsAs1DForOutWhenUnconnected=off
  B : Outport  Port=2  VectorParamsAs1DForOutWhenUnconnected=off
  C : Outport  Port=3  VectorParamsAs1DForOutWhenUnconnected=off
  wires:
  B_t/1 -> B/1, Data Type Duplicate/2
  A_t/1 -> A/1, Data Type Duplicate/1
  C_t/1 -> C/1, Data Type Duplicate/3
  Beta/1 -> Data Type Duplicate/5
  Alpha/1 -> Data Type Duplicate/4

== system Valeo_Simulink_Library_EC/Signal_Operations/VSL_InverseParkTransformation_EC_Blk/Calculation ==
  D : Inport
  sin : Inport  Port=2
  cos : Inport  Port=3
  Q : Inport  Port=4
  Add : Sum  Inputs=-+
  Add1 : Sum
  Multiply{,1..3} (4 alike) : Product  OutDataTypeStr=Inherit: Inherit via back propagation
  Alpha : Outport  VectorParamsAs1DForOutWhenUnconnected=off
  Beta : Outport  Port=2  VectorParamsAs1DForOutWhenUnconnected=off
  wires:
  Add1/1 -> Beta/1
  [d] -> Multiply/1
  Q/1 -> [q]
  D/1 -> [d]
  [d] -> Multiply2/1
  Multiply1/1 -> Add/1
  sin/1 -> Multiply1/2, Multiply/2
  Multiply/1 -> Add1/1
  cos/1 -> Multiply2/2, Multiply3/2
  Multiply2/1 -> Add/2
  Multiply3/1 -> Add1/2
  [q] -> Multiply3/1
  [q] -> Multiply1/1
  Add/1 -> Alpha/1

== system Valeo_Simulink_Library_EC/Signal_Operations/VSL_InverseParkTransformation_EC_Blk/dataTypeProtection ==
  alpha_t : Inport
  beta_t : Inport  Port=2
  D : Inport  Port=3
  Q : Inport  Port=4
  Sin : Inport  Port=5
  Cos : Inport  Port=6
  Data Type Duplicate : DataTypeDuplicate
  Data Type Duplicate1 : DataTypeDuplicate  NumInputPorts=4
  Alpha : Outport  VectorParamsAs1DForOutWhenUnconnected=off
  Beta : Outport  Port=2  VectorParamsAs1DForOutWhenUnconnected=off
  wires:
  D/1 -> Data Type Duplicate1/2
  Q/1 -> Data Type Duplicate1/3
  beta_t/1 -> Beta/1, Data Type Duplicate1/4
  Cos/1 -> Data Type Duplicate/2
  Sin/1 -> Data Type Duplicate/1
  alpha_t/1 -> Data Type Duplicate1/1, Alpha/1

== system Valeo_Simulink_Library_EC/Signal_Operations/VSL_ParkTransformation_Blk/Calculation ==
  alpha : Inport
  sin : Inport  Port=2
  cos : Inport  Port=3
  beta : Inport  Port=4
  Add : Sum  OutDataTypeStr=Inherit: Inherit via back propagation  RndMeth=Simplest
  Add1 : Sum  Inputs=-+  OutDataTypeStr=Inherit: Inherit via back propagation  RndMeth=Simplest
  Multiply{,1..3} (4 alike) : Product  OutDataTypeStr=Inherit: Inherit via back propagation  RndMeth=Simplest
  d : Outport  VectorParamsAs1DForOutWhenUnconnected=off
  q : Outport  Port=2  VectorParamsAs1DForOutWhenUnconnected=off
  wires:
  cos/1 -> Multiply2/2, Multiply3/2
  [beta] -> Multiply3/1
  sin/1 -> Multiply/2, Multiply1/2
  [alpha] -> Multiply2/1
  alpha/1 -> [alpha]
  beta/1 -> [beta]
  [alpha] -> Multiply/1
  Add/1 -> d/1
  Add1/1 -> q/1
  Multiply/1 -> Add1/1
  Multiply3/1 -> Add1/2
  Multiply1/1 -> Add/1
  Multiply2/1 -> Add/2
  [beta] -> Multiply1/1

== system Valeo_Simulink_Library_EC/Signal_Operations/VSL_ParkTransformation_Blk/DataTypeProtection ==
  d_t : Inport
  q_t : Inport  Port=2
  Alpha : Inport  Port=3
  Beta : Inport  Port=4
  Sin : Inport  Port=5
  Cos : Inport  Port=6
  Data Type Duplicate : DataTypeDuplicate  NumInputPorts=4
  Data Type Duplicate1 : DataTypeDuplicate
  D : Outport  VectorParamsAs1DForOutWhenUnconnected=off
  Q : Outport  Port=2  VectorParamsAs1DForOutWhenUnconnected=off
  wires:
  Alpha/1 -> Data Type Duplicate/2
  Beta/1 -> Data Type Duplicate/3
  q_t/1 -> Data Type Duplicate/4, Q/1
  d_t/1 -> Data Type Duplicate/1, D/1
  Sin/1 -> Data Type Duplicate1/1
  Cos/1 -> Data Type Duplicate1/2

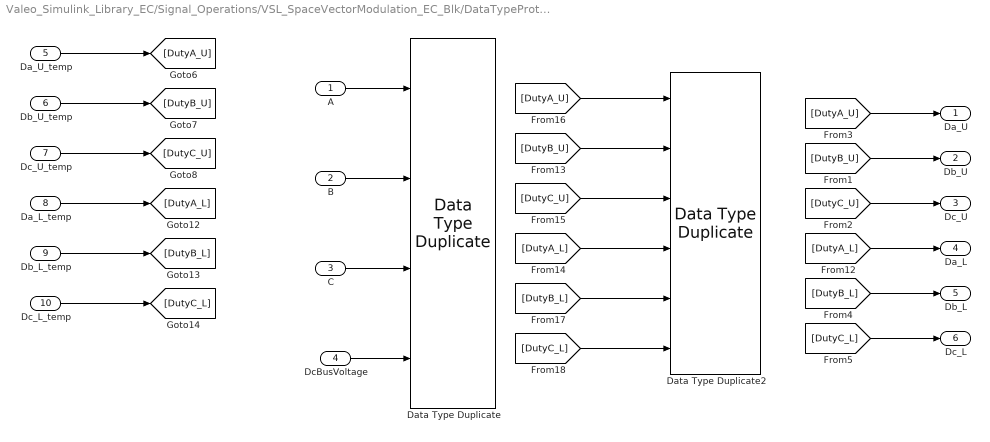
== system Valeo_Simulink_Library_EC/Signal_Operations/VSL_SpaceVectorModulation_EC_Blk/DataTypeProtection ==
  A : Inport
  B : Inport  Port=2
  C : Inport  Port=3
  DcBusVoltage : Inport  Port=4
  Da_U_temp : Inport  Port=5
  Db_U_temp : Inport  Port=6
  Dc_U_temp : Inport  Port=7
  Da_L_temp : Inport  Port=8
  Db_L_temp : Inport  Port=9
  Dc_L_temp : Inport  Port=10
  Data Type Duplicate : DataTypeDuplicate  NumInputPorts=4
  Data Type Duplicate2 : DataTypeDuplicate  NumInputPorts=6
  Da_U : Outport  VectorParamsAs1DForOutWhenUnconnected=off
  Db_U : Outport  Port=2  VectorParamsAs1DForOutWhenUnconnected=off
  Dc_U : Outport  Port=3  VectorParamsAs1DForOutWhenUnconnected=off
  Da_L : Outport  Port=4  VectorParamsAs1DForOutWhenUnconnected=off
  Db_L : Outport  Port=5  VectorParamsAs1DForOutWhenUnconnected=off
  Dc_L : Outport  Port=6  VectorParamsAs1DForOutWhenUnconnected=off
  wires:
  Db_U_temp/1 -> [DutyB_U]
  Dc_L_temp/1 -> [DutyC_L]
  Db_L_temp/1 -> [DutyB_L]
  Da_L_temp/1 -> [DutyA_L]
  Dc_U_temp/1 -> [DutyC_U]
  Da_U_temp/1 -> [DutyA_U]
  [DutyC_L] -> Data Type Duplicate2/6
  [DutyB_L] -> Data Type Duplicate2/5
  [DutyA_L] -> Data Type Duplicate2/4
  [DutyC_U] -> Data Type Duplicate2/3
  [DutyB_U] -> Data Type Duplicate2/2
  [DutyA_U] -> Data Type Duplicate2/1
  [DutyC_L] -> Dc_L/1
  [DutyB_L] -> Db_L/1
  [DutyA_L] -> Da_L/1
  A/1 -> Data Type Duplicate/1
  B/1 -> Data Type Duplicate/2
  C/1 -> Data Type Duplicate/3
  DcBusVoltage/1 -> Data Type Duplicate/4
  [DutyA_U] -> Da_U/1
  [DutyB_U] -> Db_U/1
  [DutyC_U] -> Dc_U/1

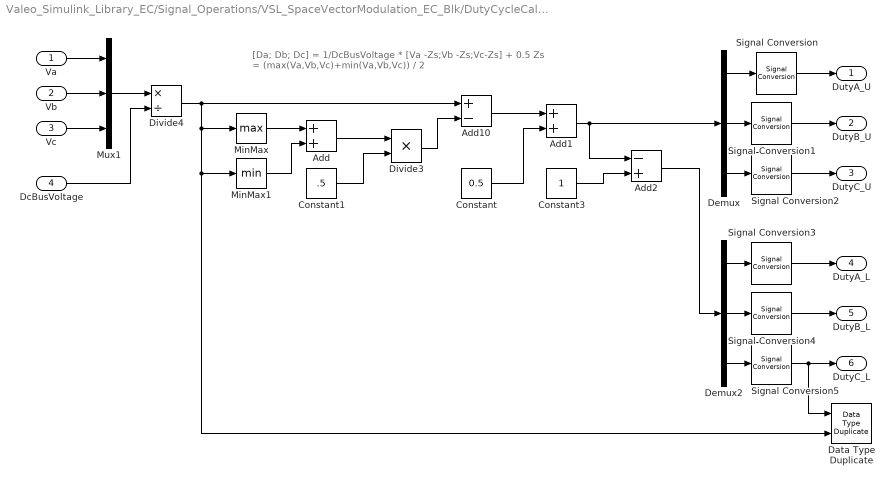
== system Valeo_Simulink_Library_EC/Signal_Operations/VSL_SpaceVectorModulation_EC_Blk/DutyCycleCalculation ==
  note: [Da; Db; Dc] = 1/DcBusVoltage * [Va -Zs;Vb -Zs;Vc-Zs] + 0.5
      | Zs = (max(Va,Vb,Vc)+min(Va,Vb,Vc)) / 2
  Va : Inport
  Vb : Inport  Port=2
  Vc : Inport  Port=3
  DcBusVoltage : Inport  Port=4
  Add : Sum  OutDataTypeStr=Inherit: Inherit via back propagation  RndMeth=Simplest
  Add1 : Sum  OutDataTypeStr=Inherit: Inherit via back propagation  RndMeth=Simplest
  Add10 : Sum  Inputs=+-  OutDataTypeStr=Inherit: Inherit via back propagation  RndMeth=Simplest
  Add2 : Sum  Inputs=-+  OutDataTypeStr=Inherit: Inherit via back propagation  RndMeth=Simplest
  Constant : Constant  Value=0.5  OutDataTypeStr=Inherit: Inherit via back propagation
  Constant1 : Constant  Value=.5  OutDataTypeStr=Inherit: Inherit via back propagation
  Constant3 : Constant  OutDataTypeStr=Inherit: Inherit via back propagation
  Data Type Duplicate : DataTypeDuplicate
  Demux : Demux  Outputs=3
  Demux2 : Demux  Outputs=3
  Divide3 : Product  Inputs=**  OutDataTypeStr=Inherit: Inherit via back propagation  RndMeth=Simplest
  Divide4 : Product  Inputs=*/  OutDataTypeStr=Inherit: Inherit via back propagation  RndMeth=Simplest
  MinMax : MinMax  Function=max  OutDataTypeStr=Inherit: Inherit via back propagation  RndMeth=Simplest
  MinMax1 : MinMax  OutDataTypeStr=Inherit: Inherit via back propagation  RndMeth=Simplest
  Mux1 : Mux  Inputs=3
  Signal Conversion{,1..5} (6 alike) : SignalConversion  OverrideOpt=off
  DutyA_U : Outport  VectorParamsAs1DForOutWhenUnconnected=off
  DutyB_U : Outport  Port=2  VectorParamsAs1DForOutWhenUnconnected=off
  DutyC_U : Outport  Port=3  VectorParamsAs1DForOutWhenUnconnected=off
  DutyA_L : Outport  Port=4  VectorParamsAs1DForOutWhenUnconnected=off
  DutyB_L : Outport  Port=5  VectorParamsAs1DForOutWhenUnconnected=off
  DutyC_L : Outport  Port=6  VectorParamsAs1DForOutWhenUnconnected=off
  wires:
  Demux2/1 -> Signal Conversion3/1
  Demux2/3 -> Signal Conversion5/1
  Demux2/2 -> Signal Conversion4/1
  Add2/1 -> Demux2/1
  Signal Conversion5/1 -> DutyC_L/1, Data Type Duplicate/1
  Signal Conversion4/1 -> DutyB_L/1
  Signal Conversion3/1 -> DutyA_L/1
  Signal Conversion2/1 -> DutyC_U/1
  Signal Conversion1/1 -> DutyB_U/1
  Signal Conversion/1 -> DutyA_U/1
  Divide4/1 -> Add10/1, MinMax/1, MinMax1/1, Data Type Duplicate/2
  DcBusVoltage/1 -> Divide4/2
  Mux1/1 -> Divide4/1
  Vc/1 -> Mux1/3
  Va/1 -> Mux1/1
  Vb/1 -> Mux1/2
  Divide3/1 -> Add10/2
  Demux/3 -> Signal Conversion2/1
  Demux/2 -> Signal Conversion1/1
  Demux/1 -> Signal Conversion/1
  Constant3/1 -> Add2/2
  Add1/1 -> Demux/1, Add2/1
  Constant/1 -> Add1/2
  Add10/1 -> Add1/1
  MinMax1/1 -> Add/2
  MinMax/1 -> Add/1
  Add/1 -> Divide3/1
  Constant1/1 -> Divide3/2

== system Valeo_Simulink_Library_EC/Utilities/EventToVar/Function-Call Subsystem ==
  in : Inport  Tag=AM,In,0,1,Name,C;CMP,Port,PortWidth,SampleTime;
  function : TriggerPort  TriggerType=function-call  VariantControl=(inherit)  StatesWhenEnabling=reset
      settings: AttributesFormatString=%<StatesWhenEnabling>
  Logical Operator1 : Logic  Tag=AM,Std,Inputs,1;CMP,Operator,Inputs;  Operator=NOT  Inputs=1  AllPortsSameDT=off  OutDataTypeStr=boolean
  out : Outport  Tag=AM,Out,1,0,Name,NC;CMP,Port,OutputWhenDisabled,InitialOutput;  InitialOutput=1  VectorParamsAs1DForOutWhenUnconnected=off
      settings: AttributesFormatString=%<OutputWhenDisabled>
  wires:
  in/1 -> Logical Operator1/1
  Logical Operator1/1 -> out/1

== system Valeo_Simulink_Library_EC/Math_Operations/VSL_DynamicSecureDivision_EC_Blk/Calculation/DecisionLogic ==
  Num : Inport  PortDimensions=1
  Den : Inport  Port=2  PortDimensions=1
  Positive_Inf : Inport  Port=3  PortDimensions=1
  Negative_Inf : Inport  Port=4  PortDimensions=1
  Nan : Inport  Port=5  PortDimensions=1
  ZeroBand_Den : Inport  Port=6  PortDimensions=1
  ZeroBand_Num : Inport  Port=7  PortDimensions=1
  DynamicSecureDivision : Stateflow chart  Description=this block is performing secure division with Positive_inf, Negative_inf, Nan is dynamic in run time  TreatAsAtomicUnit=on
  Out : Outport  VectorParamsAs1DForOutWhenUnconnected=off
  Divide : Outport  Port=2  VectorParamsAs1DForOutWhenUnconnected=off
  wires:
  ZeroBand_Num/1 -> DynamicSecureDivision/7(ZeroBand_Num)
  ZeroBand_Den/1 -> DynamicSecureDivision/6(ZeroBand_Den)
  Den/1 -> DynamicSecureDivision/2(Den)
  Num/1 -> DynamicSecureDivision/1(Num)
  Nan/1 -> DynamicSecureDivision/5(Nan)
  Positive_Inf/1 -> DynamicSecureDivision/3(Positive_Inf)
  Negative_Inf/1 -> DynamicSecureDivision/4(Negative_Inf)
  DynamicSecureDivision/2(Divide()) -> Divide/1
  DynamicSecureDivision/1(Output) -> Out/1

== system Valeo_Simulink_Library_EC/Math_Operations/VSL_DynamicSecureDivision_EC_Blk/Calculation/Divide ==
  Num : Inport
  Den : Inport  Port=2
  Trigger : TriggerPort  TriggerType=function-call  VariantControl=(inherit)
      settings: AttributesFormatString=StatesWhenEnabling: %<StatesWhenEnabling>
  Divide : Product  Inputs=*/  OutDataTypeStr=Inherit: Inherit via back propagation  RndMeth=Simplest  SaturateOnIntegerOverflow=on
  output : Outport  VectorParamsAs1DForOutWhenUnconnected=off
      settings: AttributesFormatString=OutputWhenDisabled: %<OutputWhenDisabled>
  wires:
  Divide/1 -> output/1
  Den/1 -> Divide/2
  Num/1 -> Divide/1

== system Valeo_Simulink_Library_EC/Plant Models/Actuators/BLDC/BLDC motor Block ==
  " Uab,Ubc" : Inport
  Tl : Inport  Port=2
  Add : Sum  Inputs=+-
  Demux : Demux  Outputs=5
  Electromagnetic_Torque : Subsystem
  Gain : Gain  Gain=ke/2
  Mux : Mux  Inputs=2
  Mux1 : Mux  Inputs=3
  PhaseCurrent_speed_position : StateSpace  A=[-R/L 0 0 0;0 -R/L 0 0;0 0 -kf/j 0;0 0 1 0]  B=[2/(3*L) 1/(3*L) 0;-1/(3*L) 1/(3*L) 0;0 0 1/j;0 0 0]  C=[1 0 0 0;0 1 0 0;-1 -1 0 0;0 0 1 0;0 0 0 1]  D=zeros(5,3)  InitialCondition=x0
  Product : Product
  Trapz_f : Subsystem
  Te : Outport  VectorParamsAs1DForOutWhenUnconnected=off
  Omega : Outport  Port=2  VectorParamsAs1DForOutWhenUnconnected=off
  Position : Outport  Port=3  VectorParamsAs1DForOutWhenUnconnected=off
  B_EMF : Outport  Port=4  VectorParamsAs1DForOutWhenUnconnected=off
  i_abc : Outport  Port=5  VectorParamsAs1DForOutWhenUnconnected=off
  wires:
  Demux/5 -> Trapz_f/1(Theta_m)
  Mux1/1 -> i_abc/1, Electromagnetic_Torque/2(i_abc)  "i_abc"
  Demux/1 -> Mux1/1
  Tl/1 -> Add/2
  Demux/2 -> Mux1/2
  Trapz_f/2(f_abc) -> Product/2, Electromagnetic_Torque/1(f_abc)
  Demux/3 -> Mux1/3
  Product/1 -> Gain/1
  Mux/1 -> PhaseCurrent_speed_position/1
  Demux/4 -> Omega/1, Product/1  "omega"
  " Uab,Ubc"/1 -> Mux/1
  PhaseCurrent_speed_position/1 -> Demux/1
  Trapz_f/1(Position) -> Position/1
  Electromagnetic_Torque/1(Te) -> Te/1, Add/1  "Te"
  Add/1 -> Mux/2
  Gain/1 -> B_EMF/1

== system Valeo_Simulink_Library_EC/Plant Models/Actuators/BLDC/inverter ==
  POS : Inport
  Vs : Inport  Port=2
  B_EMF : Inport  Port=3
  i_abc : Inport  Port=4
  MATLAB Function : MATLAB Function  TreatAsAtomicUnit=on
  "Uab, Ubc" : Outport  VectorParamsAs1DForOutWhenUnconnected=off
  wires:
  POS/1 -> MATLAB Function/1(POS)
  Vs/1 -> MATLAB Function/2(Vs)
  B_EMF/1 -> MATLAB Function/3(e_abc)
  i_abc/1 -> MATLAB Function/4(i_abc)
  MATLAB Function/1(U) -> "Uab, Ubc"/1

== system Valeo_Simulink_Library_EC/Signal_Operations/KalmanFilter_single/Correct/K_opt ==
  Pk_priori : Inport
  R : Inport  Port=2
  C : Inport  Port=3
  Add : Sum
  Math Function : Math  Operator=transpose  SignedPower=on  SaturateOnIntegerOverflow=on
  Matrix Divide : Product  Inputs=/  Multiplication=Matrix(*)
  Product : Product  Inputs=3  Multiplication=Matrix(*)
  Product2 : Product  Inputs=3  Multiplication=Matrix(*)
  K_optimal : Outport  VectorParamsAs1DForOutWhenUnconnected=off
  wires:
  Pk_priori/1 -> Product/1, Product2/2
  C/1 -> Product2/1, Math Function/1
  Math Function/1 -> Product/2, Product2/3
  R/1 -> Add/2
  Matrix Divide/1 -> Product/3
  Product2/1 -> Add/1
  Add/1 -> Matrix Divide/1
  Product/1 -> K_optimal/1  "K_optimal"

== system Valeo_Simulink_Library_EC/Signal_Operations/KalmanFilter_single/Correct/P_k ==
  Pk_priori : Inport
  In2 : Inport  Port=2
  R : Inport  Port=3
  C : Inport  Port=4
  Add1 : Sum
  Add4 : Sum  Inputs=+-
  Math Function1 : Math  Operator=transpose  SignedPower=on  SaturateOnIntegerOverflow=on
  Math Function2 : Math  Operator=transpose  SignedPower=on  SaturateOnIntegerOverflow=on
  Product4 : Product  Multiplication=Matrix(*)
  Product6 : Product  Inputs=3  Multiplication=Matrix(*)
  Product7 : Product  Inputs=3  Multiplication=Matrix(*)
  Var_ident_mat : Constant  Value=eye(length(A))  VectorParams1D=off  OutDataTypeStr=single
  Pk : Outport  VectorParamsAs1DForOutWhenUnconnected=off
  wires:
  C/1 -> Product4/2
  Add1/1 -> Pk/1
  Math Function2/1 -> Product7/3
  Product4/1 -> Add4/2
  In2/1 -> Math Function2/1, Product7/1, Product4/1
  Product7/1 -> Add1/2
  R/1 -> Product7/2
  Math Function1/1 -> Product6/3
  Add4/1 -> Product6/1, Math Function1/1
  Var_ident_mat/1 -> Add4/1
  Pk_priori/1 -> Product6/2
  Product6/1 -> Add1/1

== system Valeo_Simulink_Library_EC/Signal_Operations/KalmanFilter_single/Correct/X_k ==
  K_optimal : Inport
  Yk : Inport  Port=2
  Xk_priori : Inport  Port=3
  u : Inport  Port=4
  C : Inport  Port=5
  Add2 : Sum  Inputs=+--
  Add3 : Sum
  Constant2 : Constant  Value=D  VectorParams1D=off  OutDataTypeStr=single
  Product1 : Product  Multiplication=Matrix(*)
  Product3 : Product  Multiplication=Matrix(*)
  Product5 : Product  Multiplication=Matrix(*)
  Xk : Outport  OutDataTypeStr=single  InitialOutput=3  VectorParamsAs1DForOutWhenUnconnected=off
  wires:
  Product1/1 -> Add2/2
  Add3/1 -> Xk/1
  Xk_priori/1 -> Product1/2, Add3/2
  K_optimal/1 -> Product3/1
  u/1 -> Product5/2
  Yk/1 -> Add2/1
  Product5/1 -> Add2/3
  Product3/1 -> Add3/1
  Constant2/1 -> Product5/1
  Add2/1 -> Product3/2
  C/1 -> Product1/1

== system Valeo_Simulink_Library_EC/Plant Models/Actuators/BLDC/BLDC motor Block/Electromagnetic_Torque ==
  f_abc : Inport
  i_abc : Inport  Port=2
  Dot Product : DotProduct  InputSameDT=on  OutDataTypeStr=Inherit: Inherit via internal rule
  Gain : Gain  Gain=kt/2
  Te : Outport  VectorParamsAs1DForOutWhenUnconnected=off
  wires:
  f_abc/1 -> Dot Product/1
  i_abc/1 -> Dot Product/2
  Dot Product/1 -> Gain/1
  Gain/1 -> Te/1

== system Valeo_Simulink_Library_EC/Plant Models/Actuators/BLDC/BLDC motor Block/Trapz_f ==
  note: sinusoidal BEMF
  note: Instead of Position range: 0-5, output can be mapped to HALL sensor readings,
      | then inverter logic must be changed accordingly!
  Theta_m : Inport
  1-D Lookup Table : Lookup_n-D  NumberOfTableDimensions=1  BreakpointsForDimension1=0:pi/3:2*pi  Table=[1 1 1 -1 -1 -1 1]  RndMeth=Simplest  InputSameDT=on
  1-D Lookup Table1 : Lookup_n-D  NumberOfTableDimensions=1  BreakpointsForDimension1=0:pi/3:2*pi  Table=[-1 -1 1 1 1 -1 -1]  RndMeth=Simplest  InputSameDT=on
  1-D Lookup Table2 : Lookup_n-D  NumberOfTableDimensions=1  BreakpointsForDimension1=0:pi/3:2*pi  Table=[1 -1 -1 -1 1 1 1]  RndMeth=Simplest  InputSameDT=on
  1-D Lookup Table3 : Lookup_n-D  NumberOfTableDimensions=1  BreakpointsForDimension1=[0 1.047 pi/3 2.0942 2*pi/3 3.1414 pi 4.1886 4*pi/3 5.2358 5*pi/3 6.283 ]  Table=[0 0 1 1 2 2 3 3 4 4 5 5]  TableDataTypeStr=uint8  ExtrapMethod=Clip  OutDataTypeStr=uint8  RndMeth=Simplest  InputSameDT=on
  Fcn : Fcn  Expr=rem(u,2*pi)
  Gain : Gain  Gain=P/2
  Manual Switch : ManualSwitch  CurrentSetting=0
  Mux : Mux  Inputs=3
  Mux1 : Mux  Inputs=3
  Scope : Scope
  Sine Wave : Sin  TimeSource=Use external signal  SampleTime=0
  Sine Wave1 : Sin  TimeSource=Use external signal  Phase=-2*pi/3  SampleTime=0
  Sine Wave2 : Sin  TimeSource=Use external signal  Phase=-4*pi/3  SampleTime=0
  Position : Outport  VectorParamsAs1DForOutWhenUnconnected=off
  f_abc : Outport  Port=2  VectorParamsAs1DForOutWhenUnconnected=off
  wires:
  Theta_m/1 -> Gain/1
  Gain/1 -> Fcn/1
  1-D Lookup Table/1 -> Mux/1
  1-D Lookup Table1/1 -> Mux/2
  1-D Lookup Table2/1 -> Mux/3
  Mux/1 -> Manual Switch/2  "trapz"
  Fcn/1 -> 1-D Lookup Table3/1, 1-D Lookup Table2/1, 1-D Lookup Table/1, Sine Wave/1, Sine Wave1/1, Sine Wave2/1, 1-D Lookup Table1/1  "Theta_e"
  1-D Lookup Table3/1 -> Position/1
  Sine Wave2/1 -> Mux1/3
  Sine Wave1/1 -> Mux1/2
  Sine Wave/1 -> Mux1/1
  Mux1/1 -> Manual Switch/1  "sin"
  Manual Switch/1 -> Scope/1, f_abc/1
